simulink model "RollAngleHold_ModernControlS"  (R2024b)
settings: Solver=VariableStepAuto  StartTime=0.0  StopTime=25  RelTol=1e-3
values from neighbouring files (symbols this model uses):
  K = lqr(A,B,Q,R)    [PitchAttitudeHold_ModernControl.m]    (also in RollAngleHold_ModernControl.m = place(A, B, eigs))
  sysLat = ss(A,B,C,D)    [RollAngleHold_ModernControl.m]
settings Model: Creator=wangdi  LastModifiedBy=wangdi

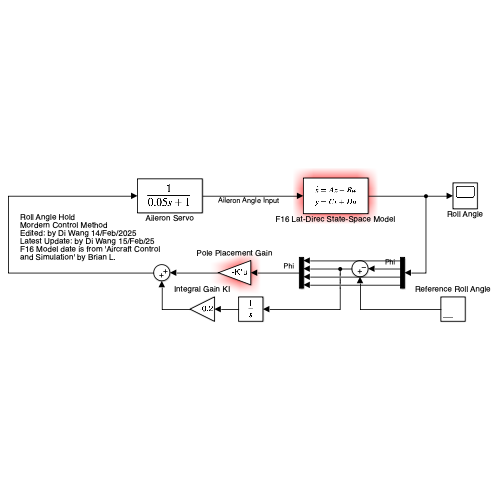
[thumbnail: Simulink's stored preview of the top-level diagram]
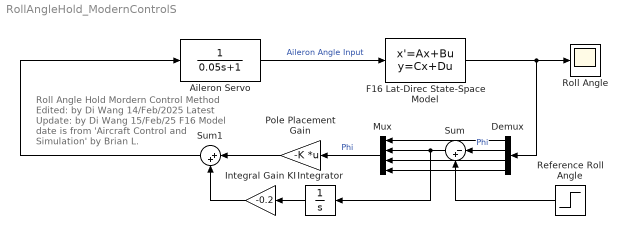
== system RollAngleHold_ModernControlS ==
  note: Roll Angle Hold
      | Mordern Control Method
      | Edited: by Di Wang 14/Feb/2025
      | Latest Update: by Di Wang 15/Feb/25
      | F16 Model date is from 'Aircraft Control and Simulation' by Brian L.
  Aileron Servo : TransferFcn  Denominator=[0.05 1]
  Demux : Demux
  F16 Lat-Direc State-Space Model : StateSpace  A=sysLat.A  B=sysLat.B  C=sysLat.C  D=sysLat.D  InitialCondition=0
  Integral Gain KI : Gain  Gain=-0.2
  Integrator : Integrator
  Mux : Mux
  Pole Placement Gain : Gain  Gain=-K  Multiplication=Matrix(K*u)
  Reference Roll Angle : Step  SampleTime=0
  Roll Angle : Scope
  Sum : Sum  Inputs=|-+
  Sum1 : Sum  Inputs=|++
  wires:
  Aileron Servo/1 -> F16 Lat-Direc State-Space Model/1  "Aileron Angle Input"
  F16 Lat-Direc State-Space Model/1 -> Roll Angle/1, Demux/1
  Demux/1 -> Mux/1
  Demux/3 -> Mux/3
  Demux/4 -> Mux/4
  Demux/2 -> Sum/1  "Phi"
  Sum/1 -> Integrator/1, Mux/2
  Reference Roll Angle/1 -> Sum/2
  Mux/1 -> Pole Placement Gain/1  "Phi"
  Sum1/1 -> Aileron Servo/1
  Pole Placement Gain/1 -> Sum1/1
  Integrator/1 -> Integral Gain KI/1
  Integral Gain KI/1 -> Sum1/2
